simulink model "gm_min_cost_function_and_vopt_FCS_MPC_6Phase_PMSM"  (R2022a)
settings: Solver=FixedStepDiscrete  StartTime=0.0  StopTime=10.0  RelTol=1e-3
undefined symbols (not defined in the file or in its folder): f_c
settings Model: Creator=Andre Merx  LastModifiedBy=Andre Merx
settings SolverCC: AlgebraicLoopSolver=TrustRegion
settings DataIOCC: LimitDataPoints=on  SaveOutput=off  SaveTime=off
settings OptimizationCC: BlockReduction=off  ConditionallyExecuteInputs=off  DefaultParameterBehavior=Inlined  LifeSpan=inf
settings DebuggingCC: AlgebraicLoopMsg=error  InheritedTsInSrcMsg=none  SingleTaskRateTransMsg=error  UnconnectedInputMsg=warning  UnconnectedOutputMsg=warning  UnconnectedLineMsg=warning  AllowSymbolicDim=off  StrictBusMsg=ErrorOnBusTreatedAsVector  SFUnexpectedBacktrackingDiag=warning  SFNoUnconditionalDefaultTransitionDiag=warning  SFExecutionAtInitializationDiag=none  SFMachineParentedDataDiag=warning  ArithmeticOperatorsInVariantConditions=warning
settings HardwareCC: ProdBitPerPointer=32  ProdBitPerSizeT=32  ProdBitPerPtrDiffT=32  ProdLargestAtomicFloat=None  ProdIntDivRoundTo=Undefined  ProdEndianess=Unspecified  ProdWordSize=32  ProdHWDeviceType=ASIC/FPGA->ASIC/FPGA  ProdEqTarget=off
settings SFSimCC: SimUseLocalCustomCode=off  CustomCodeUndefinedFunction=UseInterfaceOnly
settings RTWCC: RTWUseLocalCustomCode=off
settings CodeAppCC: StateflowObjectComments=on
settings GRTTargetCC: TargetLangStandard=C89/C90 (ANSI)
settings ConfigComp: CovScope=ReferencedModels  CovMetricSettings=dw  CovSaveCumulativeToWorkspaceVar=on  CovSaveSingleToWorkspaceVar=on  CovExternalEMLEnable=off  CovSFcnEnable=off

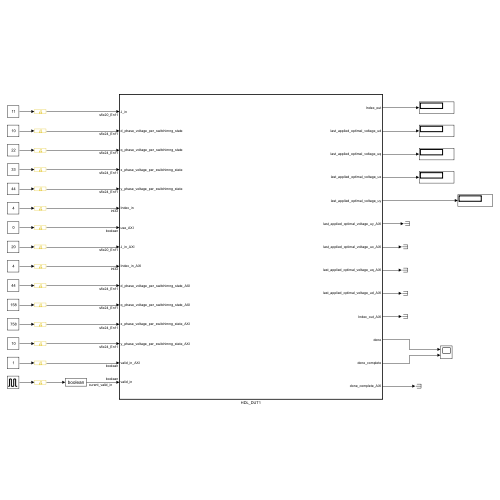
[thumbnail: Simulink's stored preview of the top-level diagram]
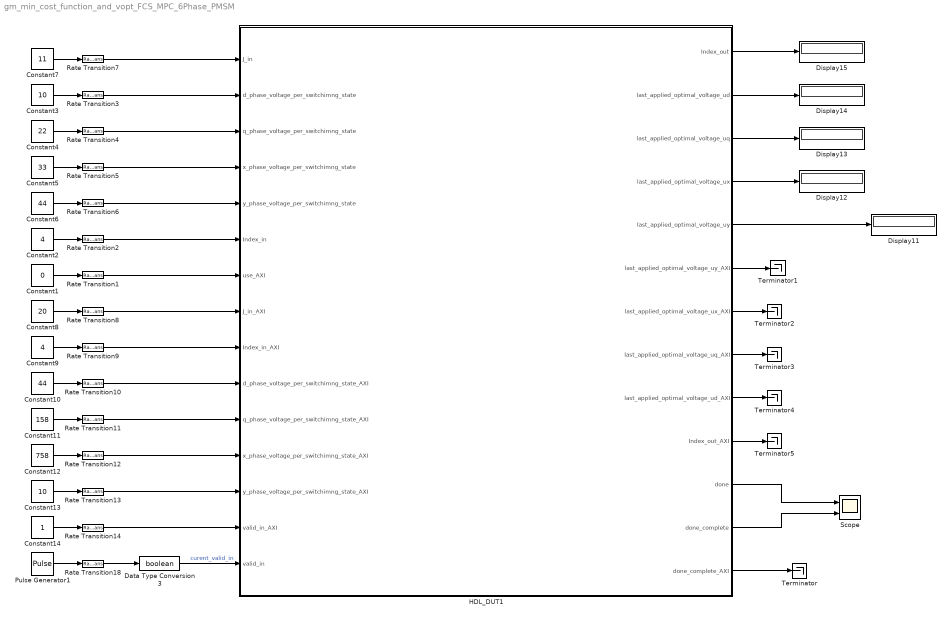
== system gm_min_cost_function_and_vopt_FCS_MPC_6Phase_PMSM ==
  Constant1 : Constant  Value=0  OutDataTypeStr=boolean  SampleTime=-1
  Constant10 : Constant  Value=44  OutDataTypeStr=fixdt(1,24,11)  SampleTime=-1  LockScale=on
  Constant11 : Constant  Value=158  OutDataTypeStr=fixdt(1,24,11)  SampleTime=-1
  Constant12 : Constant  Value=758  OutDataTypeStr=fixdt(1,24,11)  SampleTime=-1
  Constant13 : Constant  Value=10  OutDataTypeStr=fixdt(1,24,11)  SampleTime=-1
  Constant14 : Constant  OutDataTypeStr=boolean  SampleTime=-1
  Constant2 : Constant  Value=4  OutDataTypeStr=int32  SampleTime=-1
  Constant3 : Constant  Value=10  OutDataTypeStr=fixdt(1,24,11)  SampleTime=-1  LockScale=on
  Constant4 : Constant  Value=22  OutDataTypeStr=fixdt(1,24,11)  SampleTime=-1
  Constant5 : Constant  Value=33  OutDataTypeStr=fixdt(1,24,11)  SampleTime=-1
  Constant6 : Constant  Value=44  OutDataTypeStr=fixdt(1,24,11)  SampleTime=-1
  Constant7 : Constant  Value=11  OutDataTypeStr=fixdt(1,20,11)  SampleTime=-1
  Constant8 : Constant  Value=20  OutDataTypeStr=fixdt(1,20,11)  SampleTime=-1
  Constant9 : Constant  Value=4  OutDataTypeStr=int32  SampleTime=-1
  Data Type Conversion3 : DataTypeConversion  OutDataTypeStr=boolean  SaturateOnIntegerOverflow=off  RndMeth=Floor
  Display{11..15} (5 alike) : Display
  HDL_DUT1 : Subsystem  TreatAsAtomicUnit=on
  Pulse Generator1 : DiscretePulseGenerator  PulseType=Time based  Period=1/f_c
  Rate Transition{1..14,18} (15 alike) : RateTransition  OutPortSampleTime=Rt
  Scope : Scope  NumInputPorts=2
  Terminator{,1..5} (6 alike) : Terminator
  wires:
  HDL_DUT1/12(done_complete) -> Scope/2
  HDL_DUT1/11(done) -> Scope/1
  Rate Transition14/1 -> HDL_DUT1/14(valid_in_AXI)
  Constant14/1 -> Rate Transition14/1
  Rate Transition10/1 -> HDL_DUT1/10(d_phase_voltage_per_switchimng_state_AXI)
  Rate Transition11/1 -> HDL_DUT1/11(q_phase_voltage_per_switchimng_state_AXI)
  Constant10/1 -> Rate Transition10/1
  Rate Transition13/1 -> HDL_DUT1/13(y_phase_voltage_per_switchimng_state_AXI)
  Constant13/1 -> Rate Transition13/1
  Constant12/1 -> Rate Transition12/1
  Constant11/1 -> Rate Transition11/1
  Rate Transition12/1 -> HDL_DUT1/12(x_phase_voltage_per_switchimng_state_AXI)
  Rate Transition9/1 -> HDL_DUT1/9(Index_in_AXI)
  Constant9/1 -> Rate Transition9/1
  Rate Transition8/1 -> HDL_DUT1/8(J_in_AXI)
  Constant8/1 -> Rate Transition8/1
  Rate Transition1/1 -> HDL_DUT1/7(use_AXI)
  Constant1/1 -> Rate Transition1/1
  HDL_DUT1/10(Index_out_AXI) -> Terminator5/1
  HDL_DUT1/9(last_applied_optimal_voltage_ud_AXI) -> Terminator4/1
  HDL_DUT1/8(last_applied_optimal_voltage_uq_AXI) -> Terminator3/1
  HDL_DUT1/7(last_applied_optimal_voltage_ux_AXI) -> Terminator2/1
  HDL_DUT1/6(last_applied_optimal_voltage_uy_AXI) -> Terminator1/1
  HDL_DUT1/13(done_complete_AXI) -> Terminator/1
  Rate Transition7/1 -> HDL_DUT1/1(J_in)
  Constant7/1 -> Rate Transition7/1
  Rate Transition6/1 -> HDL_DUT1/5(y_phase_voltage_per_switchimng_state)
  Constant6/1 -> Rate Transition6/1
  Rate Transition5/1 -> HDL_DUT1/4(x_phase_voltage_per_switchimng_state)
  Constant5/1 -> Rate Transition5/1
  Rate Transition4/1 -> HDL_DUT1/3(q_phase_voltage_per_switchimng_state)
  Constant4/1 -> Rate Transition4/1
  Rate Transition3/1 -> HDL_DUT1/2(d_phase_voltage_per_switchimng_state)
  Constant3/1 -> Rate Transition3/1
  HDL_DUT1/1(Index_out) -> Display15/1
  HDL_DUT1/2(last_applied_optimal_voltage_ud) -> Display14/1
  HDL_DUT1/3(last_applied_optimal_voltage_uq) -> Display13/1
  HDL_DUT1/4(last_applied_optimal_voltage_ux) -> Display12/1
  HDL_DUT1/5(last_applied_optimal_voltage_uy) -> Display11/1
  Rate Transition2/1 -> HDL_DUT1/6(Index_in)
  Constant2/1 -> Rate Transition2/1
  Rate Transition18/1 -> Data Type Conversion3/1
  Pulse Generator1/1 -> Rate Transition18/1
  Data Type Conversion3/1 -> HDL_DUT1/15(valid_in)  "curent_valid_in"

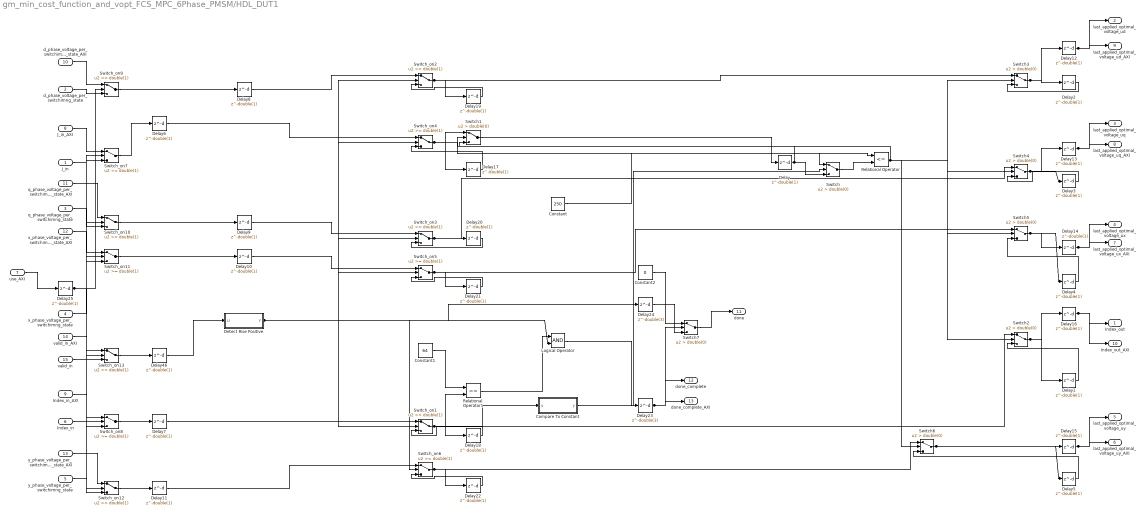
== system gm_min_cost_function_and_vopt_FCS_MPC_6Phase_PMSM/HDL_DUT1 ==
  J_in : Inport  OutDataTypeStr=fixdt(1, 20, 11)  PortDimensions=1  SampleTime=1e-08
  d_phase_voltage_per_switchimng_state : Inport  Port=2  OutDataTypeStr=fixdt(1, 24, 11)  PortDimensions=1  SampleTime=1e-08
  q_phase_voltage_per_switchimng_state : Inport  Port=3  OutDataTypeStr=fixdt(1, 24, 11)  PortDimensions=1  SampleTime=1e-08
  x_phase_voltage_per_switchimng_state : Inport  Port=4  OutDataTypeStr=fixdt(1, 24, 11)  PortDimensions=1  SampleTime=1e-08
  y_phase_voltage_per_switchimng_state : Inport  Port=5  OutDataTypeStr=fixdt(1, 24, 11)  PortDimensions=1  SampleTime=1e-08
  Index_in : Inport  Port=6  OutDataTypeStr=int32  PortDimensions=1  SampleTime=1e-08
  use_AXI : Inport  Port=7  OutDataTypeStr=boolean  PortDimensions=1  SampleTime=1e-08
  J_in_AXI : Inport  Port=8  OutDataTypeStr=fixdt(1, 20, 11)  PortDimensions=1  SampleTime=1e-08
  Index_in_AXI : Inport  Port=9  OutDataTypeStr=int32  PortDimensions=1  SampleTime=1e-08
  d_phase_voltage_per_switchimng_state_AXI : Inport  Port=10  OutDataTypeStr=fixdt(1, 24, 11)  PortDimensions=1  SampleTime=1e-08
  q_phase_voltage_per_switchimng_state_AXI : Inport  Port=11  OutDataTypeStr=fixdt(1, 24, 11)  PortDimensions=1  SampleTime=1e-08
  x_phase_voltage_per_switchimng_state_AXI : Inport  Port=12  OutDataTypeStr=fixdt(1, 24, 11)  PortDimensions=1  SampleTime=1e-08
  y_phase_voltage_per_switchimng_state_AXI : Inport  Port=13  OutDataTypeStr=fixdt(1, 24, 11)  PortDimensions=1  SampleTime=1e-08
  valid_in_AXI : Inport  Port=14  OutDataTypeStr=boolean  PortDimensions=1  SampleTime=1e-08
  valid_in : Inport  Port=15  OutDataTypeStr=boolean  PortDimensions=1  SampleTime=1e-08
  Compare To Constant : Subsystem  mask(Compare To Constant){relop=<=, const=double(1), OutDataTypeStr=boolean, ZeroCross=on}
      mask prompts: relop "Simulink:masks:Operator_MP"; const "Simulink:masks:ConstantValue_MP"; OutDataTypeStr "Simulink:masks:OutputDataType_MP"; ZeroCross "Simulink:masks:EnableZerocrossingDetection_MP"
      mask help: Simulink:masks:CompareToConstant_MD
      mask init:
      | OutDataTypeStr = 'boolean';
      | ZeroCross = 'on';
      | blkName = 'min_cost_function_and_vopt_FCS_MPC_6Phase_PMSM/HDL_DUT1/Compare\nTo Constant';
      | const = double(1);
      | const_str = '1';
      | const_val = double(1);
      | relop = '<=';
      | setValue = 'boolean';
      | str = '<= 1';
      mask TypeOptions relop: == | ~= | < | <= | >= | >
      mask TypeOptions OutDataTypeStr: Simulink:masks:uint8 | Simulink:masks:boolean
      mask Callback ZeroCross: sl('zeroCrossEnable', gcbh);
      mask Display: disp(str)
  Constant : Constant  Value=250  OutDataTypeStr=fixdt(1, 20, 11)  SampleTime=1e-08
  Constant1 : Constant  Value=64  OutDataTypeStr=int32  SampleTime=1e-08
  Constant2 : Constant  Value=0  OutDataTypeStr=boolean  SampleTime=1e-08
  Delay{,1..22,25,46} (25 alike) : Delay  DelayLength=double(1)  InitialCondition=0  SampleTime=1e-08
  Delay23 : Delay  DelayLength=double(3)  InitialCondition=0  SampleTime=1e-08
  Delay24 : Delay  DelayLength=double(3)  InitialCondition=0  SampleTime=1e-08
  Detect Rise Positive : Subsystem  mask(Detect Rise Positive){vinit=double(0), InputProcessing=Elements as channels (sample based), OutDataTypeStr=boolean}
      mask prompts: vinit "Simulink:masks:InitialCondition_MP"; InputProcessing "Simulink:masks:InputProcessing_MP"; OutDataTypeStr "Simulink:masks:OutputDataType_MP"
      mask help: Simulink:masks:DetectRisePositive_MD
      mask init:
      | InputProcessing = 'Elements as channels (sample based)';
      | OutDataTypeStr = 'boolean';
      | vinit = double(0);
      mask TypeOptions InputProcessing: Simulink:masks:ColumnsAsChannelsFrameBased | Simulink:masks:ElementsAsChannelsSampleBased
      mask TypeOptions OutDataTypeStr: Simulink:masks:uint8 | Simulink:masks:boolean
      mask Display: fprintf('U > 0\n&  NOT\nU/z > 0')
  Logical Operator : Logic  AllPortsSameDT=off  OutDataTypeStr=boolean  SampleTime=1e-08
  Relational Operator : RelationalOperator  Operator=<=  OutDataTypeStr=boolean  SampleTime=1e-08  InputSameDT=off
  Relational Operator1 : RelationalOperator  Operator===  OutDataTypeStr=boolean  SampleTime=1e-08  InputSameDT=off
  Switch : Switch  Criteria=u2 > Threshold  Threshold=double(0)  OutDataTypeStr=fixdt(1, 20, 11)  SampleTime=1e-08  SaturateOnIntegerOverflow=off  InputSameDT=off
  Switch1 : Switch  Criteria=u2 > Threshold  Threshold=double(0)  OutDataTypeStr=fixdt(1, 20, 11)  SampleTime=1e-08  SaturateOnIntegerOverflow=off  InputSameDT=off
  Switch2 : Switch  Criteria=u2 > Threshold  Threshold=double(0)  OutDataTypeStr=int32  SampleTime=1e-08  SaturateOnIntegerOverflow=off  InputSameDT=off
  Switch{3..6} (4 alike) : Switch  Criteria=u2 > Threshold  Threshold=double(0)  OutDataTypeStr=fixdt(1, 24, 11)  SampleTime=1e-08  SaturateOnIntegerOverflow=off  InputSameDT=off
  Switch7 : Switch  Criteria=u2 > Threshold  Threshold=double(0)  OutDataTypeStr=boolean  SampleTime=1e-08  SaturateOnIntegerOverflow=off  InputSameDT=off
  Switch_on1 : Switch  Threshold=double(1)  OutDataTypeStr=int32  RndMeth=Simplest  SampleTime=1e-08  SaturateOnIntegerOverflow=off  InputSameDT=off
  Switch_on{2..3,5..6,9..12} (8 alike) : Switch  Threshold=double(1)  OutDataTypeStr=fixdt(1, 24, 11)  RndMeth=Simplest  SampleTime=1e-08  SaturateOnIntegerOverflow=off  InputSameDT=off
  Switch_on13 : Switch  Threshold=double(1)  OutDataTypeStr=boolean  RndMeth=Simplest  SampleTime=1e-08  SaturateOnIntegerOverflow=off  InputSameDT=off
  Switch_on4 : Switch  Threshold=double(1)  OutDataTypeStr=fixdt(1, 20, 11)  RndMeth=Simplest  SampleTime=1e-08  SaturateOnIntegerOverflow=off  InputSameDT=off
  Switch_on7 : Switch  Threshold=double(1)  OutDataTypeStr=fixdt(1, 20, 11)  RndMeth=Simplest  SampleTime=1e-08  SaturateOnIntegerOverflow=off  InputSameDT=off
  Switch_on8 : Switch  Threshold=double(1)  OutDataTypeStr=int32  RndMeth=Simplest  SampleTime=1e-08  SaturateOnIntegerOverflow=off  InputSameDT=off
  Index_out : Outport  SampleTime=1e-08
  last_applied_optimal_voltage_ud : Outport  Port=2  SampleTime=1e-08
  last_applied_optimal_voltage_uq : Outport  Port=3  SampleTime=1e-08
  last_applied_optimal_voltage_ux : Outport  Port=4  SampleTime=1e-08
  last_applied_optimal_voltage_uy : Outport  Port=5  SampleTime=1e-08
  last_applied_optimal_voltage_uy_AXI : Outport  Port=6  SampleTime=1e-08
  last_applied_optimal_voltage_ux_AXI : Outport  Port=7  SampleTime=1e-08
  last_applied_optimal_voltage_uq_AXI : Outport  Port=8  SampleTime=1e-08
  last_applied_optimal_voltage_ud_AXI : Outport  Port=9  SampleTime=1e-08
  Index_out_AXI : Outport  Port=10  SampleTime=1e-08
  done : Outport  Port=11  SampleTime=1e-08
  done_complete : Outport  Port=12  SampleTime=1e-08
  done_complete_AXI : Outport  Port=13  SampleTime=1e-08
  wires:
  J_in/1 -> Switch_on7/3
  d_phase_voltage_per_switchimng_state/1 -> Switch_on9/3
  q_phase_voltage_per_switchimng_state/1 -> Switch_on10/3
  x_phase_voltage_per_switchimng_state/1 -> Switch_on11/3
  y_phase_voltage_per_switchimng_state/1 -> Switch_on12/3
  Index_in/1 -> Switch_on8/3
  use_AXI/1 -> Delay25/1
  J_in_AXI/1 -> Switch_on7/1
  Index_in_AXI/1 -> Switch_on8/1
  d_phase_voltage_per_switchimng_state_AXI/1 -> Switch_on9/1
  q_phase_voltage_per_switchimng_state_AXI/1 -> Switch_on10/1
  x_phase_voltage_per_switchimng_state_AXI/1 -> Switch_on11/1
  y_phase_voltage_per_switchimng_state_AXI/1 -> Switch_on12/1
  valid_in_AXI/1 -> Switch_on13/1
  valid_in/1 -> Switch_on13/3
  Compare To Constant/1(y) -> Switch/2
  Constant/1 -> Switch/1
  Constant1/1 -> Relational Operator1/1
  Constant2/1 -> Switch7/1
  Delay/1 -> Switch1/3, Switch/3
  Delay1/1 -> Switch2/3
  Delay10/1 -> Switch_on5/1
  Delay11/1 -> Switch_on6/1
  Delay12/1 -> last_applied_optimal_voltage_ud_AXI/1, last_applied_optimal_voltage_ud/1
  Delay13/1 -> last_applied_optimal_voltage_uq_AXI/1, last_applied_optimal_voltage_uq/1
  Delay14/1 -> last_applied_optimal_voltage_ux_AXI/1, last_applied_optimal_voltage_ux/1
  Delay15/1 -> last_applied_optimal_voltage_uy_AXI/1, last_applied_optimal_voltage_uy/1
  Delay16/1 -> Index_out_AXI/1, Index_out/1
  Delay17/1 -> Switch_on4/3
  Delay18/1 -> Switch_on1/3
  Delay19/1 -> Switch_on2/3
  Delay2/1 -> Switch3/3
  Delay20/1 -> Switch_on3/3
  Delay21/1 -> Switch_on5/3
  Delay22/1 -> Switch_on6/3
  Delay23/1 -> Switch7/2, done_complete_AXI/1, done_complete/1
  Delay24/1 -> Switch7/3
  Delay25/1 -> Switch_on9/2, Switch_on8/2, Switch_on7/2, Switch_on13/2, Switch_on12/2, Switch_on11/2, Switch_on10/2
  Delay3/1 -> Switch4/3
  Delay4/1 -> Switch5/3
  Delay46/1 -> Detect Rise Positive/1(U)
  Delay5/1 -> Switch6/3
  Delay6/1 -> Switch_on4/1
  Delay7/1 -> Switch_on1/1
  Delay8/1 -> Switch_on2/1
  Delay9/1 -> Switch_on3/1
  Detect Rise Positive/1(Y) -> Switch_on6/2, Switch_on5/2, Switch_on4/2, Switch_on3/2, Switch_on2/2, Switch_on1/2, Logical Operator/2, Delay24/1
  Logical Operator/1 -> Delay23/1
  Relational Operator/1 -> Switch6/2, Switch5/2, Switch4/2, Switch3/2, Switch2/2, Switch1/2
  Relational Operator1/1 -> Logical Operator/1
  Switch/1 -> Relational Operator/2
  Switch1/1 -> Delay/1
  Switch2/1 -> Delay16/1, Delay1/1
  Switch3/1 -> Delay2/1, Delay12/1
  Switch4/1 -> Delay3/1, Delay13/1
  Switch5/1 -> Delay4/1, Delay14/1
  Switch6/1 -> Delay5/1, Delay15/1
  Switch7/1 -> done/1
  Switch_on1/1 -> Switch2/1, Relational Operator1/2, Delay18/1, Compare To Constant/1(u)
  Switch_on10/1 -> Delay9/1
  Switch_on11/1 -> Delay10/1
  Switch_on12/1 -> Delay11/1
  Switch_on13/1 -> Delay46/1
  Switch_on2/1 -> Switch3/1, Delay19/1
  Switch_on3/1 -> Switch4/1, Delay20/1
  Switch_on4/1 -> Switch1/1, Relational Operator/1, Delay17/1
  Switch_on5/1 -> Switch5/1, Delay21/1
  Switch_on6/1 -> Switch6/1, Delay22/1
  Switch_on7/1 -> Delay6/1
  Switch_on8/1 -> Delay7/1
  Switch_on9/1 -> Delay8/1

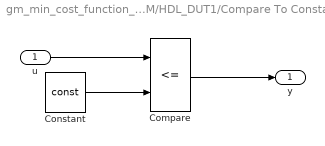
== system gm_min_cost_function_and_vopt_FCS_MPC_6Phase_PMSM/HDL_DUT1/Compare To Constant ==
  u : Inport  OutDataTypeStr=int32  SampleTime=1e-08
  Compare : RelationalOperator  Operator=<=  OutDataTypeStr=boolean
  Constant : Constant  DisableCoverage=on  Value=const  OutDataTypeStr=Inherit: Inherit via back propagation  SampleTime=-1
  y : Outport  SampleTime=1e-08
  wires:
  u/1 -> Compare/1
  Compare/1 -> y/1
  Constant/1 -> Compare/2

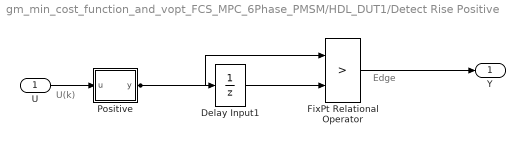
== system gm_min_cost_function_and_vopt_FCS_MPC_6Phase_PMSM/HDL_DUT1/Detect Rise Positive ==
  note: Edge
  note: U(k)
  U : Inport  OutDataTypeStr=boolean  SampleTime=1e-08
  Delay Input1 : UnitDelay  Description=Store in Global RAM  DisableCoverage=on  InitialCondition=vinit  SampleTime=-1  HasFrameUpgradeWarning=on
  FixPt Relational Operator : RelationalOperator  Operator=>  OutDataTypeStr=boolean  ZeroCross=off  InputSameDT=off
  Positive : Subsystem  mask(Compare To Zero){relop=>, OutDataTypeStr=boolean, ZeroCross=off}
      mask prompts: relop "Simulink:masks:Operator_MP"; OutDataTypeStr "Simulink:masks:OutputDataType_MP"; ZeroCross "Simulink:masks:EnableZerocrossingDetection_MP"
      mask help: Simulink:masks:CompareToZero_MD
      mask init:
      | OutDataTypeStr = 'boolean';
      | ZeroCross = 'off';
      | blkName = 'min_cost_function_and_vopt_FCS_MPC_6Phase_PMSM/HDL_DUT1/Detect Rise\nPositive/Positive';
      | relop = '>';
      | setValue = 'boolean';
      mask TypeOptions relop: == | ~= | < | <= | >= | >
      mask TypeOptions OutDataTypeStr: Simulink:masks:uint8 | Simulink:masks:boolean
      mask Callback ZeroCross: sl('zeroCrossEnable', gcbh);
      mask Display: disp([relop,' 0'])
  Y : Outport  SampleTime=1e-08
  wires:
  U/1 -> Positive/1(u)
  Delay Input1/1 -> FixPt Relational Operator/2
  FixPt Relational Operator/1 -> Y/1
  Positive/1(y) -> FixPt Relational Operator/1, Delay Input1/1

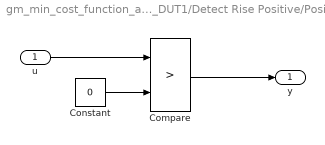
== system gm_min_cost_function_and_vopt_FCS_MPC_6Phase_PMSM/HDL_DUT1/Detect Rise Positive/Positive ==
  u : Inport  OutDataTypeStr=boolean  SampleTime=1e-08
  Compare : RelationalOperator  Operator=>  OutDataTypeStr=boolean  ZeroCross=off
  Constant : Constant  DisableCoverage=on  Value=0  OutDataTypeStr=Inherit: Inherit via back propagation  SampleTime=-1  PreserveConstantTs=on
  y : Outport  SampleTime=1e-08
  wires:
  u/1 -> Compare/1
  Compare/1 -> y/1
  Constant/1 -> Compare/2
